simulink model "ControlDelPendulo"  (R2024b)
settings: Solver=VariableStepAuto  StartTime=0.0  StopTime=10.0  RelTol=1e-3
libraries: fuzblock x1
settings Model: Creator=user  LastModifiedBy=user

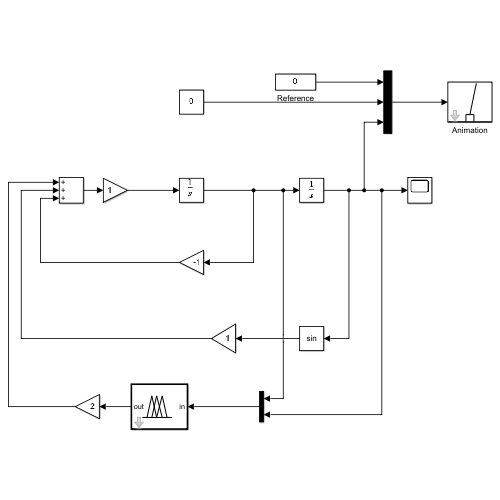
[thumbnail: Simulink's stored preview of the top-level diagram]
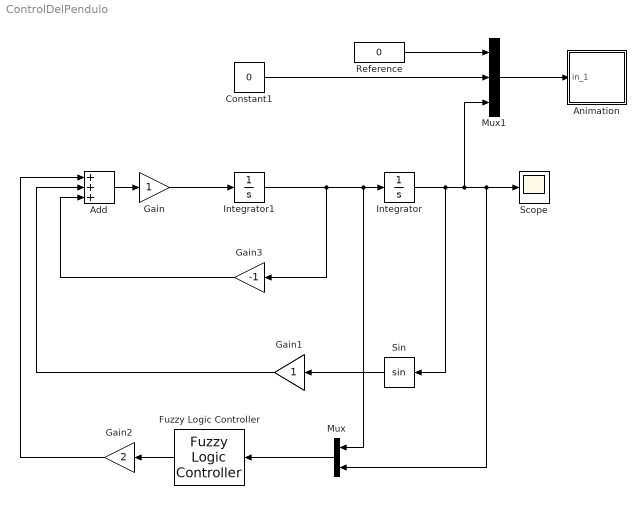
== system ControlDelPendulo ==
  Add : Sum  Inputs=+++
  Animation : Subsystem  mask(Pendulum plot){RefBlock=Reference}
      mask prompts: RefBlock "DC reference signal block name:"
      mask help: Pendulum plot
      mask Help: Pendulum animation function using Handle graphics.
      mask Display: plot([-10 10],[0 0],[-2 -2 2 2],[0 1 1 0],[0 3],[1 5])
  Constant1 : Constant  Value=0
  Fuzzy Logic Controller : fuzblock/Fuzzy Logic  Controller  FIS='ControlLogicoPendulo.fis'  OutputSampleNumber=101  DataType=double  FuzzifiedInputs=off  RuleFiringStrengths=off  RuleOutputs=off  AggregatedOutputs=off  SimulateUsing=Interpreted execution  OutOfRangeInputValueMessage=warning  NoRuleFiredMessage=warning  EmptyOutputFuzzySetMessage=warning
  Gain : Gain
  Gain1 : Gain
  Gain2 : Gain  Gain=2
  Gain3 : Gain  Gain=-1
  Integrator : Integrator  InitialCondition=pi
  Integrator1 : Integrator
  Mux : Mux  Inputs=2
  Mux1 : Mux  Inputs=3
  Reference : Constant  Value=0
  Scope : Scope
  Sin : Trigonometry
  wires:
  Integrator/1 -> Sin/1, Mux1/3, Mux/2, Scope/1
  Integrator1/1 -> Gain3/1, Mux/1, Integrator/1
  Add/1 -> Gain/1
  Gain/1 -> Integrator1/1
  Gain3/1 -> Add/3
  Sin/1 -> Gain1/1
  Gain1/1 -> Add/2
  Mux/1 -> Fuzzy Logic Controller/1
  Gain2/1 -> Add/1
  Fuzzy Logic Controller/1 -> Gain2/1
  Constant1/1 -> Mux1/2
  Mux1/1 -> Animation/1(in_1)
  Reference/1 -> Mux1/1

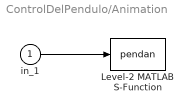
== system ControlDelPendulo/Animation ==
  in_1 : Inport
  Level-2 MATLAB S-Function : M-S-Function  FunctionName=pendan  Parameters=RefBlock
  wires:
  in_1/1 -> Level-2 MATLAB S-Function/1
